simulink model "Observador_discreto"  (R2024a)
settings: Solver=VariableStepAuto  StartTime=0.0  StopTime=10.0  RelTol=1e-3
undefined symbols (not defined in the file): A, B, C, l
settings Model: Creator=alfar  LastModifiedBy=alfar

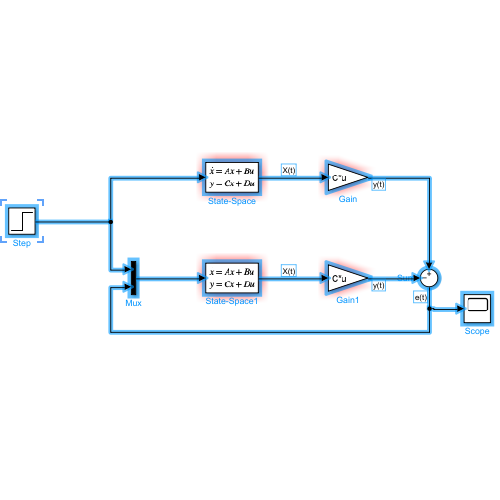
[thumbnail: Simulink's stored preview of the top-level diagram]
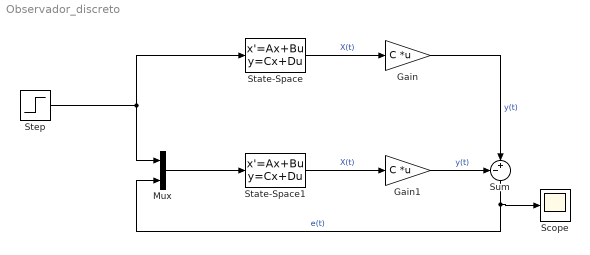
== system Observador_discreto ==
  Gain : Gain  Gain=C  Multiplication=Matrix(K*u)
  Gain1 : Gain  Gain=C  Multiplication=Matrix(K*u)
  Mux : Mux  Inputs=2
  Scope : Scope
  State-Space : StateSpace  A=A  B=B  C=eye(2)  D=zeros(2,1)  InitialCondition=0
  State-Space1 : StateSpace  A=A  B=[B l']  C=eye(2)  D=zeros(2,2)  InitialCondition=0
  Step : Step  SampleTime=0
  Sum : Sum  Inputs=-+|
  wires:
  State-Space/1 -> Gain/1  "X(t)"
  State-Space1/1 -> Gain1/1  "X(t)"
  Sum/1 -> Scope/1, Mux/2  "e(t)"
  Mux/1 -> State-Space1/1
  Gain1/1 -> Sum/1  "y(t)"
  Gain/1 -> Sum/2  "y(t)"
  Step/1 -> State-Space/1, Mux/1
